simulink model "problem4"  (R2020b)
settings: Solver=FixedStepDiscrete  StartTime=0.0  StopTime=10.0  FixedStep=0.0001  RelTol=1e-3
values from neighbouring files (symbols this model uses):
  a0 = 0.5    [Initializing.m]
  a1 = 0.25    [Initializing.m]
  b0 = 1    [Initializing.m]
  b1 = 0.4    [Initializing.m]
settings Model: Creator=Lakshmi  LastModifiedBy=Lakshmi

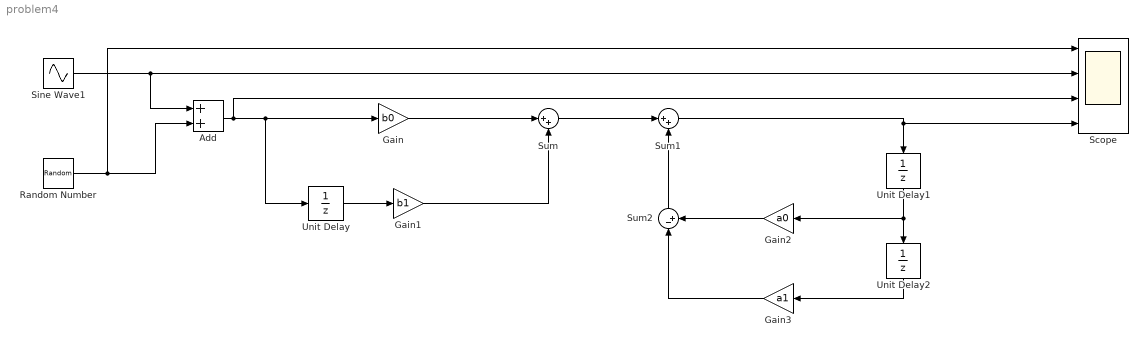
== system problem4 ==
  Add : Sum
  Gain : Gain  Gain=b0
  Gain1 : Gain  Gain=b1
  Gain2 : Gain  Gain=a0
  Gain3 : Gain  Gain=a1
  Random Number : RandomNumber  SampleTime=0.1
  Scope : Scope  NumInputPorts=4
  Sine Wave1 : Sin  Amplitude=50  SampleTime=0
  Sum : Sum  Inputs=|++
  Sum1 : Sum  Inputs=|++
  Sum2 : Sum  Inputs=|-+
  Unit Delay : UnitDelay  SampleTime=-1  HasFrameUpgradeWarning=on
  Unit Delay1 : UnitDelay  SampleTime=-1  HasFrameUpgradeWarning=on
  Unit Delay2 : UnitDelay  SampleTime=-1  HasFrameUpgradeWarning=on
  wires:
  Gain/1 -> Sum/1
  Unit Delay/1 -> Gain1/1
  Gain1/1 -> Sum/2
  Unit Delay1/1 -> Gain2/1, Unit Delay2/1
  Sum/1 -> Sum1/1
  Sum1/1 -> Unit Delay1/1, Scope/4
  Unit Delay2/1 -> Gain3/1
  Gain3/1 -> Sum2/1
  Gain2/1 -> Sum2/2
  Sum2/1 -> Sum1/2
  Random Number/1 -> Scope/1, Add/2
  Sine Wave1/1 -> Scope/2, Add/1
  Add/1 -> Scope/3, Unit Delay/1, Gain/1
